simulink model "quantizer"  (R2017a)
settings: Solver=VariableStepAuto  StartTime=0.0  StopTime=10.0  RelTol=1e-3
libraries: commsrccod2 x1
settings Model: Creator=Naveed  LastModifiedBy=Naveed

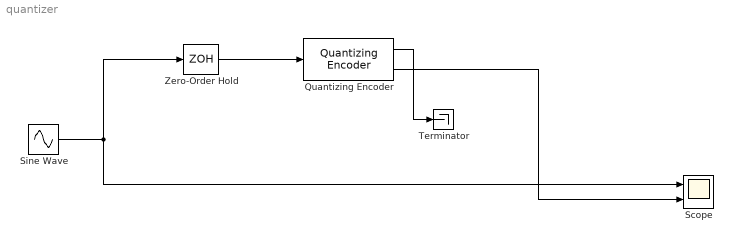
== system quantizer ==
  Quantizing Encoder : commsrccod2/Quantizing Encoder  partition=[-1:0.2:1]  codebook=[-1.1:0.2:1.1]  idxDType=double
      settings: SourceProductName=Communications System Toolbox  SourceProductBaseCode=CM
  Scope : Scope  NumInputPorts=2
  Sine Wave : Sin  SampleTime=0
  Terminator : Terminator
  Zero-Order Hold : ZeroOrderHold  SampleTime=0.1
  wires:
  Sine Wave/1 -> Zero-Order Hold/1, Scope/1
  Zero-Order Hold/1 -> Quantizing Encoder/1
  Quantizing Encoder/1 -> Terminator/1
  Quantizing Encoder/2 -> Scope/2
